simulink model "SIL_PIL"  (R2023b)
settings: Solver=FixedStepDiscrete  StartTime=0.0  StopTime=10.0  FixedStep=Ts  RelTol=1e-3  EnableMultiTasking=on
values from neighbouring files (symbols this model uses):
  kr = -1/(C*inv(A-B*K_tilde(1:3))*B)    [controller_tuning.m]    (also in progetto.m = -1/(C*inv(A-B*K)*B); tuning.m)
  num_int = -num{1}    [controller_tuning.m]
  sys_discrete = c2d(sys_continuos,0.005,'tustin')    [observer.m]
  Ts = 0.005    [attempt.m]    (also in model_approximation.m; tuning.m)
undefined symbols (not defined in the file or in its folder): K_tilde
settings Model: ExtModeTrigDuration=10  Creator=giova  LastModifiedBy=david
settings OptimizationCC: EnhancedBackFolding=on  PassReuseOutputArgsAs=Individual arguments  ZeroExternalMemoryAtStartup=off  ZeroInternalMemoryAtStartup=off  MaxStackSize=64  OptimizeBlockOrder=speed  DifferentSizesBufferReuse=on  OptimizationCustomize=off  EfficientTunableParamExpr=on
settings DebuggingCC: ParameterTunabilityLossMsg=error
settings HardwareCC: ProdBitPerPointer=32  ProdBitPerSizeT=32  ProdBitPerPtrDiffT=32  ProdLargestAtomicInteger=Long  ProdLargestAtomicFloat=Double  ProdWordSize=32  ProdLongLongMode=on  ProdHWDeviceType=ARM Compatible->ARM Cortex
settings SFSimCC: MATLABDynamicMemAlloc=off
settings RTWCC: Description=Embedded Coder  SystemTargetFile=ert.tlc  HardwareBoard=STM32 Nucleo F401RE  TemplateMakefile=ert_default_tmf  Toolchain=GNU Tools for ARM Embedded Processors  PortableWordSizes=on
settings CodeAppCC: ForceParamTrailComments=on  IgnoreCustomStorageClasses=off  OperatorAnnotations=on  SimulinkDataObjDesc=on  SFDataObjDesc=on  InsertBlockDesc=on
settings ERTTargetCC: ExtModeTransport=3  ExtModeStaticAlloc=on  ExtModeStaticAllocSize=2000  ExtModeMexFile=ext_xcp  ExtModeIntrfLevel=Level2 - Open

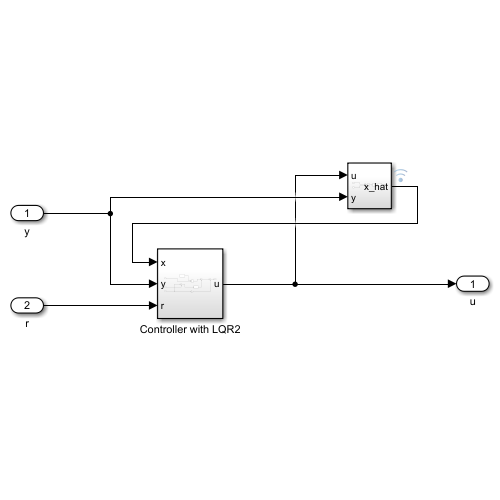
[thumbnail: Simulink's stored preview of the top-level diagram]
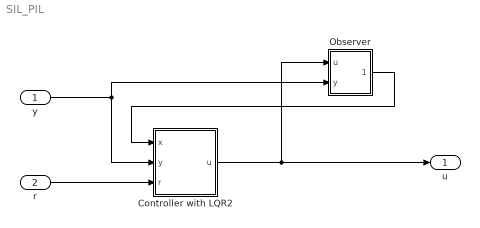
== system SIL_PIL ==
  y : Inport
  r : Inport  Port=2
  Controller with LQR2 : Subsystem
  Observer : Subsystem
  u : Outport
  wires:
  y/1 -> Controller with LQR2/2(y), Observer/2(y)
  r/1 -> Controller with LQR2/3(r)
  Controller with LQR2/1(u) -> u/1, Observer/1(u)
  Observer/1(x_hat) -> Controller with LQR2/1(x)

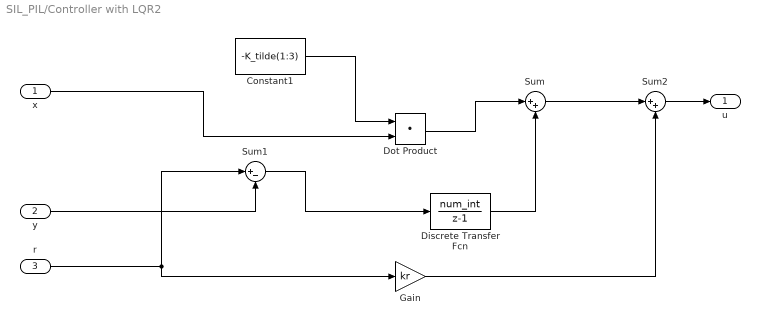
== system SIL_PIL/Controller with LQR2 ==
  x : Inport
  y : Inport  Port=2
  r : Inport  Port=3
  Constant1 : Constant  Value=-K_tilde(1:3)
  Discrete Transfer Fcn : DiscreteTransferFcn  Numerator=num_int  Denominator=[1 -1]  SampleTime=Ts  StateName='slowIntState'
  Dot Product : DotProduct  OutDataTypeStr=Inherit: Inherit via internal rule
  Gain : Gain  Gain=kr
  Sum : Sum  Inputs=|++
  Sum1 : Sum  Inputs=|+-
  Sum2 : Sum  Inputs=|++
  u : Outport
  wires:
  Dot Product/1 -> Sum/1
  Discrete Transfer Fcn/1 -> Sum/2
  Sum1/1 -> Discrete Transfer Fcn/1
  y/1 -> Sum1/2
  x/1 -> Dot Product/2
  Sum2/1 -> u/1
  Constant1/1 -> Dot Product/1
  Sum/1 -> Sum2/1
  r/1 -> Gain/1, Sum1/1
  Gain/1 -> Sum2/2

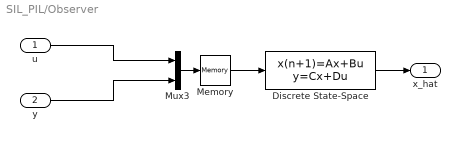
== system SIL_PIL/Observer ==
  u : Inport
  y : Inport  Port=2
  Discrete State-Space : DiscreteStateSpace  A=sys_discrete.A  B=sys_discrete.B  C=sys_discrete.C  D=sys_discrete.D  SampleTime=Ts
  Memory : Memory
  Mux3 : Mux  Inputs=2
  x_hat : Outport
  wires:
  y/1 -> Mux3/2
  u/1 -> Mux3/1
  Mux3/1 -> Memory/1
  Discrete State-Space/1 -> x_hat/1
  Memory/1 -> Discrete State-Space/1
